simulink model "NUgus_IK"  (R2018a)
settings: Solver=VariableStepAuto  StartTime=0.0  StopTime=inf  RelTol=1e-3
values from neighbouring files (symbols this model uses):
  CM740_acc_bias = 4 * 9.80743    (= 39.22972)    [CM740_init.m]
  CM740_acc_gain = 512 / CM740_acc_centre    [CM740_init.m]
  CM740_gyro_bias = 1600 / 360 * 2 * pi    (= 27.9252680319)    [CM740_init.m]
  CM740_gyro_gain = 512 / CM740_gyro_centre    [CM740_init.m]
  head = [-0.05482228998067195, -0.00010888238321339966, 0.0011712900228573724, 0.41900000000000004]    [comtest.m]
  s = mean(abs(present_speed.data))    [RunServoTest.m]
  torso = [0.0050079703254699804, 0.008880921777563762, 0.1021503146237477, 2.5390000000000006]    [comtest.m]
undefined symbols (not defined in the file or in its folder): floor, X, Y, Z
libraries: sm_lib x211, fl_lib x128, nesl_utility x68
(part 1 of 8)
settings Model: Creator=matt  LastModifiedBy=matt
settings DebuggingCC: UniqueDataStoreMsg=error
settings ExplorerConfigSet: InternalSimMechanicsExplorerSettings="<ExplorerConfiguration><canonicalview>default</canonicalview><AnimationSetting><BasePlaybackSpeed>1.0</BasePlaybackSpeed><PlaybackSpeedFactor>0.125</PlaybackSpeedFactor></AnimationSetting><TilePanel><TileInfo><Tiles Columns=\"1\" Count=\"1\" Rows=\"1\"><Column Weight=\"1\"/><Row Weight=\"1\"/><Tile Height=\"1\" Width=\"1\" X=\"0\" Y=\"0\"/></Tiles></TileInfo><SceneInfo><SceneViewer><BGColor><R>0.800000011920928955</R><G>0.800000011920928955</G><B>0.800000011920928955</B></BGColor><Camera><DoPerspective>off</DoPerspective><Position><X>0.996097398048217064</X><Y>-0.871904325438711214</Y><Z>0.621451067428618886</Z></Position><Center><X>-0.122665475521987533</X><Y>0.224636309977359006</Y><Z>0.297935636755597033</Z></Center><Up><X>-0.160360573572373266</X><Y>0.125250173842771817</Y><Z>0.97907960881426559</Z></Up><ViewLimDist>1</ViewLimDist><YLim>0.594254607494361209</YLim><XLim>0.353738210919678941</XLim></Camera></SceneViewer></SceneInfo></TilePanel><MechEditorPanel><Cameras/><GfxPanelCameraMap/><VideoCreator><PlaybackSpeedRatio>1.0</PlaybackSpeedRatio><FrameRate>30</FrameRate><VideoFormat>Motion JPEG AVI</VideoFormat><FrameSize>auto</FrameSize></VideoCreator></MechEditorPanel></ExplorerConfiguration>"

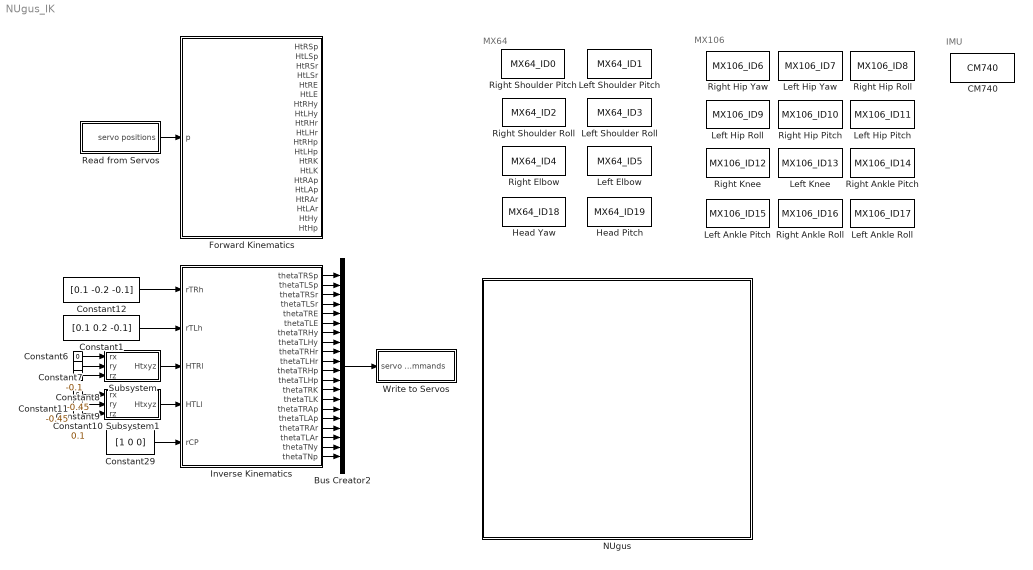
== system NUgus_IK ==
  note: IMU
  note: MX64
  note: MX106
  Bus Creator2 : BusCreator  Inputs=20
  CM740 : DataStoreMemory  DataStoreName=CM740  ReadBeforeWriteMsg=warning  WriteAfterWriteMsg=warning  WriteAfterReadMsg=warning  InitialValue=CM740_default  VectorParams1D=off  ShowAdditionalParam=off  OutDataTypeStr=Bus: CM740_bus
  Constant1 : Constant  Value=[0.1 0.2 -0.1]
  Constant10 : Constant  Value=0.1
  Constant11 : Constant  Value=-0.45
  Constant12 : Constant  Value=[0.1 -0.2 -0.1]
  Constant29 : Constant  Value=[1 0 0]
  Constant6 : Constant  Value=0
  Constant7 : Constant  Value=-0.1
  Constant8 : Constant  Value=-0.45
  Constant9 : Constant  Value=0
  Forward Kinematics : Subsystem
  Head Pitch : DataStoreMemory  DataStoreName=MX64_ID19  ReadBeforeWriteMsg=warning  WriteAfterWriteMsg=warning  WriteAfterReadMsg=warning  InitialValue=MX64_default  VectorParams1D=off  ShowAdditionalParam=off  OutDataTypeStr=Bus: MX64_bus
  Head Yaw : DataStoreMemory  DataStoreName=MX64_ID18  ReadBeforeWriteMsg=warning  WriteAfterWriteMsg=warning  WriteAfterReadMsg=warning  InitialValue=MX64_default  VectorParams1D=off  ShowAdditionalParam=off  OutDataTypeStr=Bus: MX64_bus
  Inverse Kinematics : Subsystem
  Left Ankle Pitch : DataStoreMemory  DataStoreName=MX106_ID15  ReadBeforeWriteMsg=warning  WriteAfterWriteMsg=warning  WriteAfterReadMsg=warning  InitialValue=MX106_default  VectorParams1D=off  ShowAdditionalParam=off  OutDataTypeStr=Bus: MX106_bus
  Left Ankle Roll : DataStoreMemory  DataStoreName=MX106_ID17  ReadBeforeWriteMsg=warning  WriteAfterWriteMsg=warning  WriteAfterReadMsg=warning  InitialValue=MX106_default  VectorParams1D=off  ShowAdditionalParam=off  OutDataTypeStr=Bus: MX106_bus
  Left Elbow : DataStoreMemory  DataStoreName=MX64_ID5  ReadBeforeWriteMsg=warning  WriteAfterWriteMsg=warning  WriteAfterReadMsg=warning  InitialValue=MX64_default  VectorParams1D=off  ShowAdditionalParam=off  OutDataTypeStr=Bus: MX64_bus
  Left Hip Pitch : DataStoreMemory  DataStoreName=MX106_ID11  ReadBeforeWriteMsg=warning  WriteAfterWriteMsg=warning  WriteAfterReadMsg=warning  InitialValue=MX106_default  VectorParams1D=off  ShowAdditionalParam=off  OutDataTypeStr=Bus: MX106_bus
  Left Hip Roll : DataStoreMemory  DataStoreName=MX106_ID9  ReadBeforeWriteMsg=warning  WriteAfterWriteMsg=warning  WriteAfterReadMsg=warning  InitialValue=MX106_default  VectorParams1D=off  ShowAdditionalParam=off  OutDataTypeStr=Bus: MX106_bus
  Left Hip Yaw : DataStoreMemory  DataStoreName=MX106_ID7  ReadBeforeWriteMsg=warning  WriteAfterWriteMsg=warning  WriteAfterReadMsg=warning  InitialValue=MX106_default  VectorParams1D=off  ShowAdditionalParam=off  OutDataTypeStr=Bus: MX106_bus
  Left Knee : DataStoreMemory  DataStoreName=MX106_ID13  ReadBeforeWriteMsg=warning  WriteAfterWriteMsg=warning  WriteAfterReadMsg=warning  InitialValue=MX106_default  VectorParams1D=off  ShowAdditionalParam=off  OutDataTypeStr=Bus: MX106_bus
  Left Shoulder Pitch : DataStoreMemory  DataStoreName=MX64_ID1  ReadBeforeWriteMsg=warning  WriteAfterWriteMsg=warning  WriteAfterReadMsg=warning  InitialValue=MX64_default  VectorParams1D=off  ShowAdditionalParam=off  OutDataTypeStr=Bus: MX64_bus
  Left Shoulder Roll : DataStoreMemory  DataStoreName=MX64_ID3  ReadBeforeWriteMsg=warning  WriteAfterWriteMsg=warning  WriteAfterReadMsg=warning  InitialValue=MX64_default  VectorParams1D=off  ShowAdditionalParam=off  OutDataTypeStr=Bus: MX64_bus
  NUgus : Subsystem
      mask Display: image('./img/NUgus.png');
  Read from Servos : Subsystem
  Right Ankle Pitch : DataStoreMemory  DataStoreName=MX106_ID14  ReadBeforeWriteMsg=warning  WriteAfterWriteMsg=warning  WriteAfterReadMsg=warning  InitialValue=MX106_default  VectorParams1D=off  ShowAdditionalParam=off  OutDataTypeStr=Bus: MX106_bus
  Right Ankle Roll : DataStoreMemory  DataStoreName=MX106_ID16  ReadBeforeWriteMsg=warning  WriteAfterWriteMsg=warning  WriteAfterReadMsg=warning  InitialValue=MX106_default  VectorParams1D=off  ShowAdditionalParam=off  OutDataTypeStr=Bus: MX106_bus
  Right Elbow : DataStoreMemory  DataStoreName=MX64_ID4  ReadBeforeWriteMsg=warning  WriteAfterWriteMsg=warning  WriteAfterReadMsg=warning  InitialValue=MX64_default  VectorParams1D=off  ShowAdditionalParam=off  OutDataTypeStr=Bus: MX64_bus
  Right Hip Pitch : DataStoreMemory  DataStoreName=MX106_ID10  ReadBeforeWriteMsg=warning  WriteAfterWriteMsg=warning  WriteAfterReadMsg=warning  InitialValue=MX106_default  VectorParams1D=off  ShowAdditionalParam=off  OutDataTypeStr=Bus: MX106_bus
  Right Hip Roll : DataStoreMemory  DataStoreName=MX106_ID8  ReadBeforeWriteMsg=warning  WriteAfterWriteMsg=warning  WriteAfterReadMsg=warning  InitialValue=MX106_default  VectorParams1D=off  ShowAdditionalParam=off  OutDataTypeStr=Bus: MX106_bus
  Right Hip Yaw : DataStoreMemory  DataStoreName=MX106_ID6  InitialValue=MX106_default  VectorParams1D=off  ShowAdditionalParam=off  OutDataTypeStr=Bus: MX106_bus
  Right Knee : DataStoreMemory  DataStoreName=MX106_ID12  ReadBeforeWriteMsg=warning  WriteAfterWriteMsg=warning  WriteAfterReadMsg=warning  InitialValue=MX106_default  VectorParams1D=off  ShowAdditionalParam=off  OutDataTypeStr=Bus: MX106_bus
  Right Shoulder Pitch : DataStoreMemory  DataStoreName=MX64_ID0  ReadBeforeWriteMsg=warning  WriteAfterWriteMsg=warning  WriteAfterReadMsg=warning  InitialValue=MX64_default  VectorParams1D=off  ShowAdditionalParam=off  OutDataTypeStr=Bus: MX64_bus
  Right Shoulder Roll : DataStoreMemory  DataStoreName=MX64_ID2  ReadBeforeWriteMsg=warning  WriteAfterWriteMsg=warning  WriteAfterReadMsg=warning  InitialValue=MX64_default  VectorParams1D=off  ShowAdditionalParam=off  OutDataTypeStr=Bus: MX64_bus
  Subsystem : Subsystem
  Subsystem1 : Subsystem
  Write to Servos : Subsystem
  wires:
  Inverse Kinematics/1(thetaTRSp) -> Bus Creator2/1
  Inverse Kinematics/2(thetaTLSp) -> Bus Creator2/2
  Inverse Kinematics/3(thetaTRSr) -> Bus Creator2/3
  Inverse Kinematics/4(thetaTLSr) -> Bus Creator2/4
  Inverse Kinematics/5(thetaTRE) -> Bus Creator2/5
  Inverse Kinematics/6(thetaTLE) -> Bus Creator2/6
  Inverse Kinematics/7(thetaTRHy) -> Bus Creator2/7
  Inverse Kinematics/8(thetaTLHy) -> Bus Creator2/8
  Inverse Kinematics/9(thetaTRHr) -> Bus Creator2/9
  Inverse Kinematics/10(thetaTLHr) -> Bus Creator2/10
  Inverse Kinematics/11(thetaTRHp) -> Bus Creator2/11
  Inverse Kinematics/12(thetaTLHp) -> Bus Creator2/12
  Inverse Kinematics/13(thetaTRK) -> Bus Creator2/13
  Inverse Kinematics/14(thetaTLK) -> Bus Creator2/14
  Inverse Kinematics/15(thetaTRAp) -> Bus Creator2/15
  Inverse Kinematics/16(thetaTLAp) -> Bus Creator2/16
  Inverse Kinematics/17(thetaTRAr) -> Bus Creator2/17
  Inverse Kinematics/18(thetaTLAr) -> Bus Creator2/18
  Inverse Kinematics/19(thetaTNy) -> Bus Creator2/19
  Inverse Kinematics/20(thetaTNp) -> Bus Creator2/20
  Bus Creator2/1 -> Write to Servos/1(servo commands)
  Constant12/1 -> Inverse Kinematics/1(rTRh)
  Constant1/1 -> Inverse Kinematics/2(rTLh)
  Constant29/1 -> Inverse Kinematics/5(rCP)
  Constant7/1 -> Subsystem/2(ry)
  Constant8/1 -> Subsystem/3(rz)
  Constant6/1 -> Subsystem/1(rx)
  Subsystem/1(Htxyz) -> Inverse Kinematics/3(HTRl)
  Constant11/1 -> Subsystem1/3(rz)
  Constant9/1 -> Subsystem1/1(rx)
  Constant10/1 -> Subsystem1/2(ry)
  Subsystem1/1(Htxyz) -> Inverse Kinematics/4(HTLl)
  Read from Servos/1(servo positions) -> Forward Kinematics/1(p)

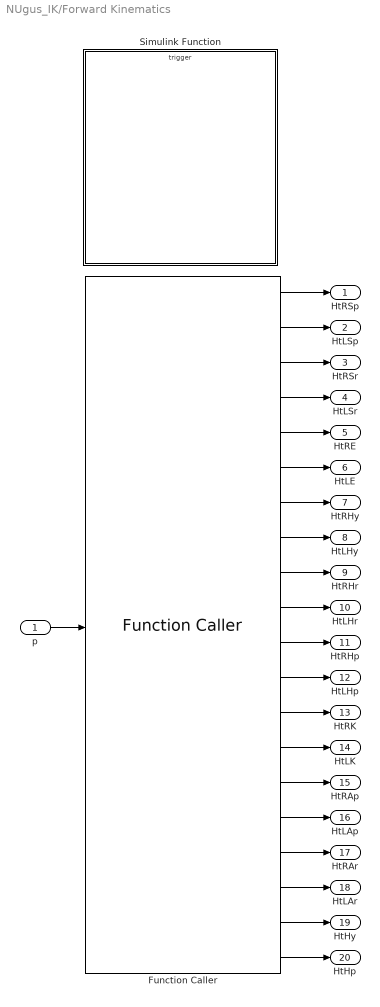
== system NUgus_IK/Forward Kinematics ==
  p : Inport
  Function Caller : FunctionCaller  FunctionPrototype=[HtRSp,HtLSp,HtRSr,HtLSr,HtRE,HtLE,HtRHy,HtLHy,HtRHr,HtLHr,HtRHp,HtLHp,HtRK,HtLK,HtRAp,HtLAp,HtRAr,HtLAr,HtHy,HtHp] = FK(p)  InputArgumentSpecifications=double([1 1 1 1 1 1 1 1 1 1 1 1 1 1 1 1 1 1 1 1])
  Simulink Function : Subsystem  TreatAsAtomicUnit=on
  HtRSp : Outport
  HtLSp : Outport  Port=2
  HtRSr : Outport  Port=3
  HtLSr : Outport  Port=4
  HtRE : Outport  Port=5
  HtLE : Outport  Port=6
  HtRHy : Outport  Port=7
  HtLHy : Outport  Port=8
  HtRHr : Outport  Port=9
  HtLHr : Outport  Port=10
  HtRHp : Outport  Port=11
  HtLHp : Outport  Port=12
  HtRK : Outport  Port=13
  HtLK : Outport  Port=14
  HtRAp : Outport  Port=15
  HtLAp : Outport  Port=16
  HtRAr : Outport  Port=17
  HtLAr : Outport  Port=18
  HtHy : Outport  Port=19
  HtHp : Outport  Port=20
  wires:
  Function Caller/2 -> HtLSp/1
  Function Caller/1 -> HtRSp/1
  Function Caller/3 -> HtRSr/1
  Function Caller/4 -> HtLSr/1
  Function Caller/5 -> HtRE/1
  Function Caller/6 -> HtLE/1
  Function Caller/7 -> HtRHy/1
  Function Caller/8 -> HtLHy/1
  Function Caller/9 -> HtRHr/1
  Function Caller/10 -> HtLHr/1
  Function Caller/11 -> HtRHp/1
  Function Caller/12 -> HtLHp/1
  Function Caller/13 -> HtRK/1
  Function Caller/14 -> HtLK/1
  Function Caller/15 -> HtRAp/1
  Function Caller/16 -> HtLAp/1
  Function Caller/17 -> HtRAr/1
  Function Caller/18 -> HtLAr/1
  Function Caller/19 -> HtHy/1
  Function Caller/20 -> HtHp/1
  p/1 -> Function Caller/1

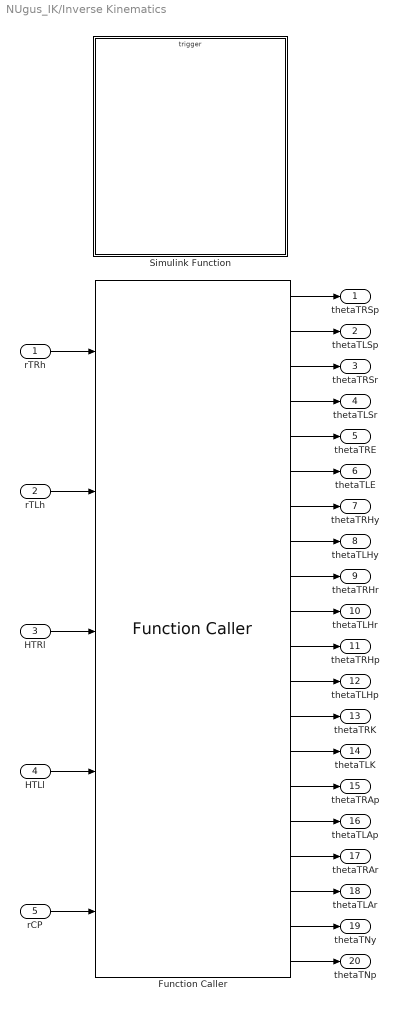
== system NUgus_IK/Inverse Kinematics ==
  rTRh : Inport
  rTLh : Inport  Port=2
  HTRl : Inport  Port=3
  HTLl : Inport  Port=4
  rCP : Inport  Port=5
  Function Caller : FunctionCaller  FunctionPrototype=[thetaTRSp,thetaTLSp,thetaTRSr,thetaTLSr,thetaTRE,thetaTLE,thetaTRHy,thetaTLHy,thetaTRHr,thetaTLHr,thetaTRHp,thetaTLHp,thetaTRK,thetaTLK,thetaTRAp,thetaTLAp,thetaTRAr,thetaTLAr,thetaTNy,thetaTNp] = IK(rTRh,rTLh,HTRl,HTLl,rCP)
  Simulink Function : Subsystem  TreatAsAtomicUnit=on
  thetaTRSp : Outport
  thetaTLSp : Outport  Port=2
  thetaTRSr : Outport  Port=3
  thetaTLSr : Outport  Port=4
  thetaTRE : Outport  Port=5
  thetaTLE : Outport  Port=6
  thetaTRHy : Outport  Port=7
  thetaTLHy : Outport  Port=8
  thetaTRHr : Outport  Port=9
  thetaTLHr : Outport  Port=10
  thetaTRHp : Outport  Port=11
  thetaTLHp : Outport  Port=12
  thetaTRK : Outport  Port=13
  thetaTLK : Outport  Port=14
  thetaTRAp : Outport  Port=15
  thetaTLAp : Outport  Port=16
  thetaTRAr : Outport  Port=17
  thetaTLAr : Outport  Port=18
  thetaTNy : Outport  Port=19
  thetaTNp : Outport  Port=20
  wires:
  Function Caller/2 -> thetaTLSp/1
  Function Caller/1 -> thetaTRSp/1
  Function Caller/3 -> thetaTRSr/1
  Function Caller/4 -> thetaTLSr/1
  Function Caller/5 -> thetaTRE/1
  Function Caller/6 -> thetaTLE/1
  Function Caller/7 -> thetaTRHy/1
  Function Caller/8 -> thetaTLHy/1
  Function Caller/9 -> thetaTRHr/1
  Function Caller/10 -> thetaTLHr/1
  Function Caller/11 -> thetaTRHp/1
  Function Caller/12 -> thetaTLHp/1
  Function Caller/13 -> thetaTRK/1
  Function Caller/14 -> thetaTLK/1
  Function Caller/15 -> thetaTRAp/1
  Function Caller/16 -> thetaTLAp/1
  Function Caller/17 -> thetaTRAr/1
  Function Caller/18 -> thetaTLAr/1
  Function Caller/19 -> thetaTNy/1
  Function Caller/20 -> thetaTNp/1
  rTRh/1 -> Function Caller/1
  rTLh/1 -> Function Caller/2
  HTRl/1 -> Function Caller/3
  HTLl/1 -> Function Caller/4
  rCP/1 -> Function Caller/5

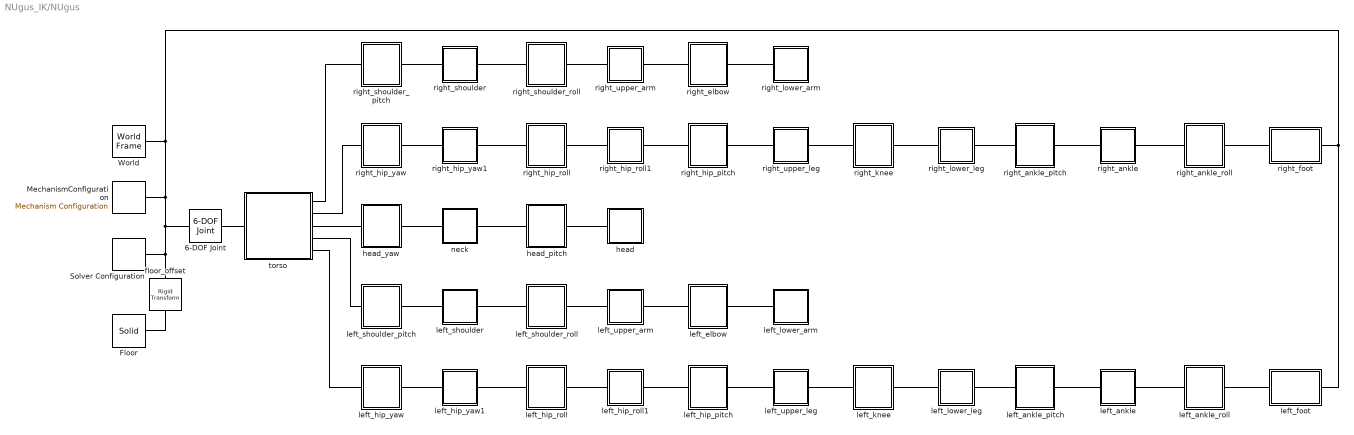
== system NUgus_IK/NUgus ==
  6-DOF Joint : sm_lib/Joints/6-DOF Joint  SenseConstraintForce=off  SenseConstraintForceX=off  SenseConstraintForceY=off  SenseConstraintForceZ=off  SenseConstraintTorque=off  SenseConstraintTorqueX=off  SenseConstraintTorqueY=off  SenseConstraintTorqueZ=off  SenseTotalForce=off  SenseTotalForceX=off  SenseTotalForceY=off  SenseTotalForceZ=off  SenseTotalTorque=off  SenseTotalTorqueX=off  SenseTotalTorqueY=off  SenseTotalTorqueZ=off  CompositeWrenchDir=FollowerOnBase  CompositeWrenchFrame=BaseFrame  PxEquilibriumPosition=0  PxEquilibriumPositionUnits=m  PxSpringStiffness=0  PxSpringStiffnessUnits=N/m  PxDampingCoefficient=0  PxDampingCoefficientUnits=N/(m/s)  PxTorqueActuationMode=NoTorque  PxMotionActuationMode=ComputedMotion  PxSensePosition=off  PxSenseVelocity=off  PxSenseAcceleration=off  PxSenseTorqueForce=off  PxPositionTargetSpecify=off  PxPositionTargetPriority=High  PxPositionTargetValue=0  PxPositionTargetValueUnits=m  PxVelocityTargetSpecify=off  PxVelocityTargetPriority=High  PxVelocityTargetValue=0  PxVelocityTargetValueUnits=m/s  PyEquilibriumPosition=0  PyEquilibriumPositionUnits=m  PySpringStiffness=0  PySpringStiffnessUnits=N/m  PyDampingCoefficient=0  PyDampingCoefficientUnits=N/(m/s)  PyTorqueActuationMode=NoTorque  PyMotionActuationMode=ComputedMotion  PySensePosition=off  PySenseVelocity=off  PySenseAcceleration=off  PySenseTorqueForce=off  PyPositionTargetSpecify=off  PyPositionTargetPriority=High  PyPositionTargetValue=0  PyPositionTargetValueUnits=m  PyVelocityTargetSpecify=off  PyVelocityTargetPriority=High  PyVelocityTargetValue=0  PyVelocityTargetValueUnits=m/s  PzEquilibriumPosition=0  PzEquilibriumPositionUnits=m  PzSpringStiffness=0  PzSpringStiffnessUnits=N/m  PzDampingCoefficient=0  PzDampingCoefficientUnits=N/(m/s)  PzTorqueActuationMode=NoTorque  PzMotionActuationMode=ComputedMotion  PzSensePosition=off  PzSenseVelocity=off  PzSenseAcceleration=off  PzSenseTorqueForce=off  PzPositionTargetSpecify=on  PzPositionTargetPriority=High  PzPositionTargetValue=0.52+floor.depth  PzPositionTargetValueUnits=m  PzVelocityTargetSpecify=off  PzVelocityTargetPriority=High  PzVelocityTargetValue=0  PzVelocityTargetValueUnits=m/s  SphDefPosRotationMethod=None  SphDefPosRotationAngleUnits=deg  SphDefPosRotationStandardAxis=+Z  SphDefPosRotationAngle=0.0  SphDefPosRotationArbitraryAxis=[0 0 1]  SphDefPosFollAlignAxisA=+X  SphDefPosBaseAlignAxisA=+Y  SphDefPosFollAlignAxisB=+Y  SphDefPosBaseAlignAxisB=+Z  SphDefPosRotationSequenceAxes=FollowerAxes  SphDefPosRotationSequence=XYX  SphDefPosRotationSequenceAngles=[0 0 0]  SphDefPosRotationSequenceAnglesUnits=deg  SphDefPosRotationMatrix=[1 0 0; 0 1 0; 0 0 1]  SphEqPosRotationMethod=None  SphEqPosRotationAngleUnits=deg  SphEqPosRotationStandardAxis=+Z  SphEqPosRotationAngle=0.0  SphEqPosRotationArbitraryAxis=[0 0 1]  SphEqPosFollAlignAxisA=+X  SphEqPosBaseAlignAxisA=+Y  SphEqPosFollAlignAxisB=+Y  SphEqPosBaseAlignAxisB=+Z  SphEqPosRotationSequenceAxes=FollowerAxes  SphEqPosRotationSequence=XYX  SphEqPosRotationSequenceAngles=[0 0 0]  SphEqPosRotationSequenceAnglesUnits=deg  SphEqPosRotationMatrix=[1 0 0; 0 1 0; 0 0 1]  SphSpringStiffness=0  SphSpringStiffnessUnits=N*m/deg  SphDampingCoefficient=0  SphDampingCoefficientUnits=N*m/(deg/s)  SphActuateTorqueX=off  SphActuateTorqueY=off  SphActuateTorqueZ=off  SphActuateTorque=off  SphTorqueActuationMode=NoTorque  SphMotionActuationMode=ComputedMotion  SphActuationFrame=BaseFrame  SphSensePosition=off  SphSenseVelocityX=off  SphSenseVelocityY=off  SphSenseVelocityZ=off  SphSenseVelocity=off  SphSenseAccelerationX=off  SphSenseAccelerationY=off  SphSenseAccelerationZ=off  SphSenseAcceleration=off  SphSenseTorqueX=off  SphSenseTorqueY=off  SphSenseTorqueZ=off  SphSenseTorqueForce=off  SphSensingFrame=BaseFrame  SphPositionTargetRotationMethod=None  SphPositionTargetRotationAngleUnits=deg  SphPositionTargetRotationStandardAxis=+Z  SphPositionTargetRotationAngle=0.0  SphPositionTargetRotationArbitraryAxis=[0 0 1]  SphPositionTargetFollAlignAxisA=+X  SphPositionTargetBaseAlignAxisA=+Y  SphPositionTargetFollAlignAxisB=+Y  SphPositionTargetBaseAlignAxisB=+Z  SphPositionTargetRotationSequenceAxes=FollowerAxes  SphPositionTargetRotationSequence=XYX  SphPositionTargetRotationSequenceAngles=[0 0 0]  SphPositionTargetRotationSequenceAnglesUnits=deg  SphPositionTargetRotationMatrix=[1 0 0; 0 1 0; 0 0 1]  SphPositionTargetSpecify=off  SphPositionTargetPriority=High  SphVelocityTargetValue=[0 0 0]  SphVelocityTargetValueUnits=deg/s  SphVelocityTargetSpecify=off  SphVelocityTargetPriority=High  SphVelocityTargetInFollowerFrame=on
  Floor : sm_lib/Body Elements/Solid  InertiaType=CalculateFromGeometry  Mass=1  MassUnits=kg  CenterOfMass=[0 0 0]  CenterOfMassUnits=m  MomentsOfInertia=[1 1 1]  MomentsOfInertiaUnits=kg*m^2  ProductsOfInertia=[0 0 0]  ProductsOfInertiaUnits=kg*m^2  DensityBased=on  Density=1000  DensityUnits=kg/m^3  DoExposeReferenceFrame=on  SerializedFrames=<Frames/>  GraphicType=FromGeometry  MarkerShape=Frame  MarkerSize=10  GraphicVisPropType=SimpleVisualProperties  GraphicDiffuseColor=[0.972549 0.972549 0.972549]  GraphicSpecularColor=[0.3 0.3 0.3 1.0]  GraphicAmbientColor=[0.20 0.20 0.20 1.0]  GraphicEmissiveColor=[0.0 0.0 0.0 1.0]  GraphicShininess=30  GraphicOpacity=0.6  GeometryShape=Brick  RectangleSize=[1 1]  RectangleSizeUnits=m  BrickDimensions=[floor.length floor.width floor.depth]  BrickDimensionUnits=m  CylinderRadius=1  CylinderRadiusUnits=m  CylinderLength=1  CylinderLengthUnits=m  SphereRadius=1  SphereRadiusUnits=m  EllipsoidRadii=[1 1 1]  EllipsoidRadiiUnits=m  ExtrusionCrossSection=[1 1; -1 1; -1 -1; 1 -1]  ExtrusionCrossSectionUnits=m  ExtrusionLength=1  ExtrusionLengthUnits=m  PolygonNumSides=3  PolygonOuterRadius=1  PolygonOuterRadiusUnits=m  ExtGeomFileType=STEP  ExtGeomFileUnits=m  RevolutionCrossSection=[1 1; 1 -1; 2 -1; 2 1]  RevolutionCrossSectionUnits=m  RevolutionExtent=Full  RevolutionAngle=180  RevolutionAngleUnits=deg
  MechanismConfiguration : sm_lib/Utilities/Mechanism Configuration  UniformGravity=Constant  GravityVector=[0 0 -9.80665]  GravityUnits=m/s^2  LinearizationDelta=0.001
  Solver Configuration : nesl_utility/Solver Configuration  PhysicalDomain=network_engine_domain  SubClassName=solver  LeftPortType=input  RightPortType=generic  Tones=[]  Harmonics=[]  SimulateNoise=off  Profile=off  UseLocalSampling=off  EnableSwitchedLinearOptims=on  FrequencyDomain=off  UseCCode=off  RelTol=0.001  AbsTol=1e-06  MinStep=1e-09  ToWorkspace=off  RevertToSquareIcSolve=off  NumHomotopyIterations=100  PhasorMode=off  PhasorModeNumHarmonics=1  DoDC=off  ResidualTolerance=1e-09  UseLocalSolver=off  LocalSolverChoice=NE_BACKWARD_EULER_ADVANCER  LocalSolverSampleTime=0.001  DoFixedCost=off  MaxNonlinIter=3  MaxModeIter=2  LinearAlgebra=Sparse  EquationFormulation=NE_TIME_EF  DelaysMemoryBudget=1024  AutomaticFiltering=on  FilteringTimeConstant=0.001
  World : sm_lib/Frames and Transforms/World Frame
  floor_offset : sm_lib/Frames and Transforms/Rigid Transform  TranslationMethod=Cartesian  TranslationStandardOffset=0  TranslationLengthUnit=m  TranslationStandardAxis=+Z  TranslationCartesianOffset=[0 0 floor.depth/2]  TranslationROffset=0  TranslationROffsetUnits=m  TranslationZOffset=0  TranslationZOffsetUnits=m  TranslationThetaOffset=0  TranslationThetaOffsetUnits=deg  RotationMethod=None  RotationAngleUnits=deg  RotationStandardAxis=+Z  RotationAngle=0.0  RotationArbitraryAxis=[0 0 1]  FollAlignAxisA=+X  BaseAlignAxisA=+Y  FollAlignAxisB=+Y  BaseAlignAxisB=+Z  RotationSequenceAxes=FollowerAxes  RotationSequence=XYX  RotationSequenceAngles=[0 0 0]  RotationSequenceAnglesUnits=deg  RotationMatrix=[1 0 0; 0 1 0; 0 0 1]
  head : Subsystem
  head_pitch : Subsystem
      mask Display: image('./img/MX64.png');
  head_yaw : Subsystem
      mask Display: image('./img/MX64.png');
  left_ankle : Subsystem
  left_ankle_pitch : Subsystem
      mask Display: image('./img/MX106.png');
  left_ankle_roll : Subsystem
      mask Display: image('./img/MX106.png');
  left_elbow : Subsystem
      mask Display: image('./img/MX64.png');
  left_foot : Subsystem
  left_hip_pitch : Subsystem
      mask Display: image('./img/MX106.png');
  left_hip_roll : Subsystem
      mask Display: image('./img/MX106.png');
  left_hip_roll1 : Subsystem
  left_hip_yaw : Subsystem
      mask Display: image('./img/MX106.png');
  left_hip_yaw1 : Subsystem
  left_knee : Subsystem
      mask Display: image('./img/MX106.png');
  left_lower_arm : Subsystem
  left_lower_leg : Subsystem
  left_shoulder : Subsystem
  left_shoulder_pitch : Subsystem
      mask Display: image('./img/MX64.png');
  left_shoulder_roll : Subsystem
      mask Display: image('./img/MX64.png');
  left_upper_arm : Subsystem
  left_upper_leg : Subsystem
  neck : Subsystem
  right_ankle : Subsystem
  right_ankle_pitch : Subsystem
      mask Display: image('./img/MX106.png');
  right_ankle_roll : Subsystem
      mask Display: image('./img/MX106.png');
  right_elbow : Subsystem
      mask Display: image('./img/MX64.png');
  right_foot : Subsystem
  right_hip_pitch : Subsystem
      mask Display: image('./img/MX106.png');
  right_hip_roll : Subsystem
      mask Display: image('./img/MX106.png');
  right_hip_roll1 : Subsystem
  right_hip_yaw : Subsystem
      mask Display: image('./img/MX106.png');
  right_hip_yaw1 : Subsystem
  right_knee : Subsystem
      mask Display: image('./img/MX106.png');
  right_lower_arm : Subsystem
  right_lower_leg : Subsystem
  right_shoulder : Subsystem
  right_shoulder_pitch : Subsystem
      mask Display: image('./img/MX64.png');
  right_shoulder_roll : Subsystem
      mask Display: image('./img/MX64.png');
  right_upper_arm : Subsystem
  right_upper_leg : Subsystem
  torso : Subsystem
  connections:
  right_ankle_roll/LConn1 -- right_ankle/RConn1
  left_elbow/RConn1 -- left_lower_arm/LConn1
  left_knee/RConn1 -- left_lower_leg/LConn1
  left_hip_roll/LConn1 -- left_hip_yaw1/RConn1
  left_hip_yaw/RConn1 -- left_hip_yaw1/LConn1
  torso/RConn3 -- head_yaw/LConn1
  right_shoulder_roll/LConn1 -- right_shoulder/RConn1
  right_hip_pitch/LConn1 -- right_hip_roll1/RConn1
  right_hip_yaw1/RConn1 -- right_hip_roll/LConn1
  head_pitch/LConn1 -- neck/RConn1
  6-DOF Joint/RConn1 -- torso/LConn1
  Floor/RConn1 -- floor_offset/RConn1
  right_lower_arm/LConn1 -- right_elbow/RConn1
  head/LConn1 -- head_pitch/RConn1
  left_shoulder/RConn1 -- left_shoulder_roll/LConn1
  left_hip_pitch/RConn1 -- left_upper_leg/LConn1
  left_foot/LConn1 -- left_ankle_roll/RConn1
  torso/RConn1 -- right_shoulder_pitch/LConn1
  right_hip_pitch/RConn1 -- right_upper_leg/LConn1
  right_hip_yaw/LConn1 -- torso/RConn2
  left_shoulder_pitch/LConn1 -- torso/RConn4
  left_ankle_pitch/RConn1 -- left_ankle/LConn1
  left_ankle_pitch/LConn1 -- left_lower_leg/RConn1
  left_knee/LConn1 -- left_upper_leg/RConn1
  left_hip_roll/RConn1 -- left_hip_roll1/LConn1
  MechanismConfiguration/RConn1 -- left_foot/RConn1 -- right_foot/RConn1 -- World/RConn1 -- 6-DOF Joint/LConn1 -- floor_offset/LConn1 -- Solver Configuration/RConn1
  left_upper_arm/LConn1 -- left_shoulder_roll/RConn1
  left_shoulder_pitch/RConn1 -- left_shoulder/LConn1
  left_ankle_roll/LConn1 -- left_ankle/RConn1
  right_ankle_pitch/RConn1 -- right_ankle/LConn1
  right_ankle_pitch/LConn1 -- right_lower_leg/RConn1
  neck/LConn1 -- head_yaw/RConn1
  right_knee/RConn1 -- right_lower_leg/LConn1
  right_ankle_roll/RConn1 -- right_foot/LConn1
  right_knee/LConn1 -- right_upper_leg/RConn1
  right_hip_roll1/LConn1 -- right_hip_roll/RConn1
  right_shoulder_pitch/RConn1 -- right_shoulder/LConn1
  right_elbow/LConn1 -- right_upper_arm/RConn1
  right_hip_yaw/RConn1 -- right_hip_yaw1/LConn1
  left_elbow/LConn1 -- left_upper_arm/RConn1
  left_hip_roll1/RConn1 -- left_hip_pitch/LConn1
  torso/RConn5 -- left_hip_yaw/LConn1
  right_shoulder_roll/RConn1 -- right_upper_arm/LConn1

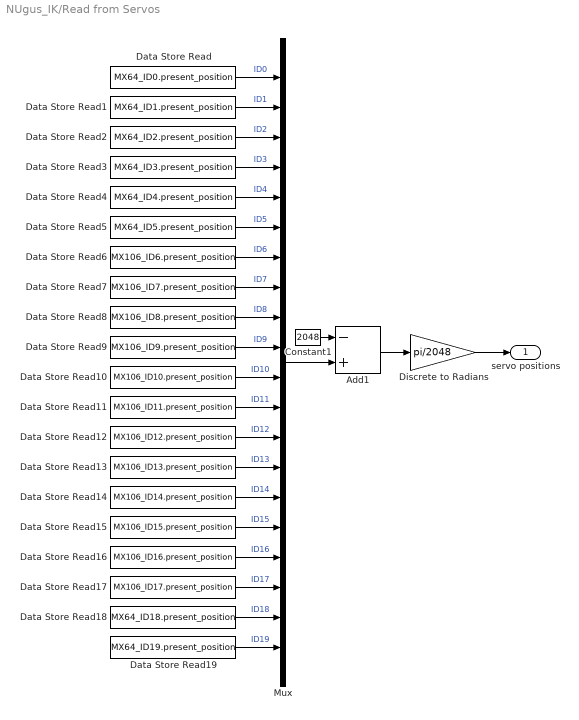
== system NUgus_IK/Read from Servos ==
  Add1 : Sum  Inputs=-+  OutDataTypeStr=double
  Constant1 : Constant  Value=2048
  Data Store Read : DataStoreRead  DataStoreName=MX64_ID0  DataStoreElements=MX64_ID0.present_position
  Data Store Read1 : DataStoreRead  DataStoreName=MX64_ID1  DataStoreElements=MX64_ID1.present_position
  Data Store Read10 : DataStoreRead  DataStoreName=MX106_ID10  DataStoreElements=MX106_ID10.present_position
  Data Store Read11 : DataStoreRead  DataStoreName=MX106_ID11  DataStoreElements=MX106_ID11.present_position
  Data Store Read12 : DataStoreRead  DataStoreName=MX106_ID12  DataStoreElements=MX106_ID12.present_position
  Data Store Read13 : DataStoreRead  DataStoreName=MX106_ID13  DataStoreElements=MX106_ID13.present_position
  Data Store Read14 : DataStoreRead  DataStoreName=MX106_ID14  DataStoreElements=MX106_ID14.present_position
  Data Store Read15 : DataStoreRead  DataStoreName=MX106_ID15  DataStoreElements=MX106_ID15.present_position
  Data Store Read16 : DataStoreRead  DataStoreName=MX106_ID16  DataStoreElements=MX106_ID16.present_position
  Data Store Read17 : DataStoreRead  DataStoreName=MX106_ID17  DataStoreElements=MX106_ID17.present_position
  Data Store Read18 : DataStoreRead  DataStoreName=MX64_ID18  DataStoreElements=MX64_ID18.present_position
  Data Store Read19 : DataStoreRead  DataStoreName=MX64_ID19  DataStoreElements=MX64_ID19.present_position
  Data Store Read2 : DataStoreRead  DataStoreName=MX64_ID2  DataStoreElements=MX64_ID2.present_position
  Data Store Read3 : DataStoreRead  DataStoreName=MX64_ID3  DataStoreElements=MX64_ID3.present_position
  Data Store Read4 : DataStoreRead  DataStoreName=MX64_ID4  DataStoreElements=MX64_ID4.present_position
  Data Store Read5 : DataStoreRead  DataStoreName=MX64_ID5  DataStoreElements=MX64_ID5.present_position
  Data Store Read6 : DataStoreRead  DataStoreName=MX106_ID6  DataStoreElements=MX106_ID6.present_position
  Data Store Read7 : DataStoreRead  DataStoreName=MX106_ID7  DataStoreElements=MX106_ID7.present_position
  Data Store Read8 : DataStoreRead  DataStoreName=MX106_ID8  DataStoreElements=MX106_ID8.present_position
  Data Store Read9 : DataStoreRead  DataStoreName=MX106_ID9  DataStoreElements=MX106_ID9.present_position
  Discrete to Radians : Gain  Gain=pi/2048  SaturateOnIntegerOverflow=on  OutDataTypeStr=Inherit: Same as input
  Mux : Mux  Inputs=20
  servo positions : Outport  PortDimensions=20
  wires:
  Data Store Read19/1 -> Mux/20  "ID19"
  Data Store Read18/1 -> Mux/19  "ID18"
  Data Store Read17/1 -> Mux/18  "ID17"
  Data Store Read/1 -> Mux/1  "ID0"
  Data Store Read1/1 -> Mux/2  "ID1"
  Data Store Read2/1 -> Mux/3  "ID2"
  Data Store Read3/1 -> Mux/4  "ID3"
  Data Store Read4/1 -> Mux/5  "ID4"
  Data Store Read5/1 -> Mux/6  "ID5"
  Data Store Read6/1 -> Mux/7  "ID6"
  Data Store Read7/1 -> Mux/8  "ID7"
  Data Store Read8/1 -> Mux/9  "ID8"
  Data Store Read9/1 -> Mux/10  "ID9"
  Data Store Read10/1 -> Mux/11  "ID10"
  Data Store Read11/1 -> Mux/12  "ID11"
  Data Store Read12/1 -> Mux/13  "ID12"
  Data Store Read13/1 -> Mux/14  "ID13"
  Data Store Read14/1 -> Mux/15  "ID14"
  Data Store Read15/1 -> Mux/16  "ID15"
  Data Store Read16/1 -> Mux/17  "ID16"
  Mux/1 -> Add1/2
  Constant1/1 -> Add1/1
  Add1/1 -> Discrete to Radians/1
  Discrete to Radians/1 -> servo positions/1

== system NUgus_IK/Subsystem ==
  rx : Inport
  ry : Inport  Port=2
  rz : Inport  Port=3
  Bus Creator3 : BusCreator  Inputs=4
  Bus to Vector2 : BusToVector
  Constant : Constant
  Constant9 : Constant  Value=[1 0 0; 0 1 0; 0 0 1; 0 0 0]
  Matrix Concatenate : Concatenate  Mode=Multidimensional array  ConcatenateDimension=2
  Htxyz : Outport
  wires:
  Bus to Vector2/1 -> Matrix Concatenate/2
  ry/1 -> Bus Creator3/2
  Bus Creator3/1 -> Bus to Vector2/1
  Matrix Concatenate/1 -> Htxyz/1
  rx/1 -> Bus Creator3/1
  rz/1 -> Bus Creator3/3
  Constant9/1 -> Matrix Concatenate/1
  Constant/1 -> Bus Creator3/4

== system NUgus_IK/Subsystem1 ==
  rx : Inport
  ry : Inport  Port=2
  rz : Inport  Port=3
  Bus Creator3 : BusCreator  Inputs=4
  Bus to Vector2 : BusToVector
  Constant : Constant
  Constant9 : Constant  Value=[1 0 0; 0 1 0; 0 0 1; 0 0 0]
  Matrix Concatenate : Concatenate  Mode=Multidimensional array  ConcatenateDimension=2
  Htxyz : Outport
  wires:
  Bus to Vector2/1 -> Matrix Concatenate/2
  ry/1 -> Bus Creator3/2
  Bus Creator3/1 -> Bus to Vector2/1
  Matrix Concatenate/1 -> Htxyz/1
  rx/1 -> Bus Creator3/1
  rz/1 -> Bus Creator3/3
  Constant9/1 -> Matrix Concatenate/1
  Constant/1 -> Bus Creator3/4

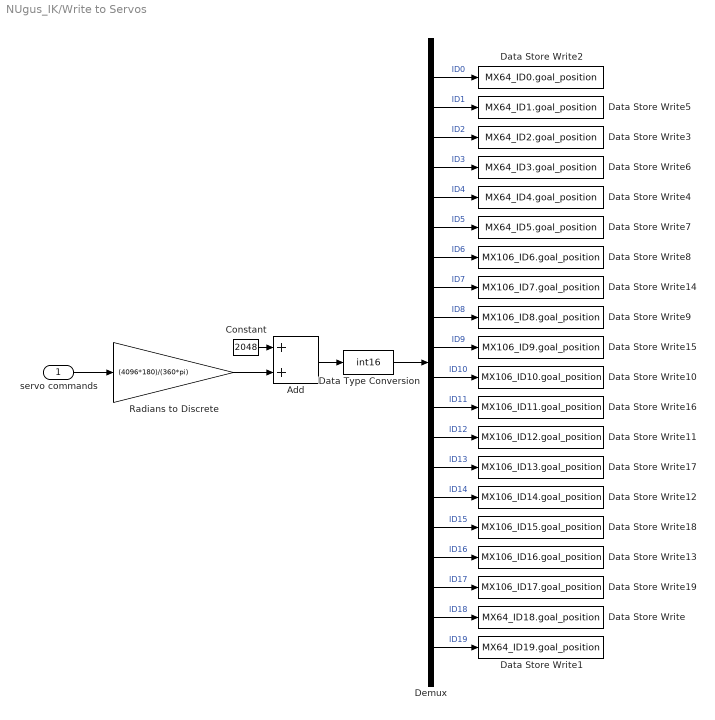
== system NUgus_IK/Write to Servos ==
  servo commands : Inport  PortDimensions=20
  Add : Sum
  Constant : Constant  Value=2048
  Data Store Write : DataStoreWrite  DataStoreName=MX64_ID18  DataStoreElements=MX64_ID18.goal_position
  Data Store Write1 : DataStoreWrite  DataStoreName=MX64_ID19  DataStoreElements=MX64_ID19.goal_position
  Data Store Write10 : DataStoreWrite  DataStoreName=MX106_ID10  DataStoreElements=MX106_ID10.goal_position
  Data Store Write11 : DataStoreWrite  DataStoreName=MX106_ID12  DataStoreElements=MX106_ID12.goal_position
  Data Store Write12 : DataStoreWrite  DataStoreName=MX106_ID14  DataStoreElements=MX106_ID14.goal_position
  Data Store Write13 : DataStoreWrite  DataStoreName=MX106_ID16  DataStoreElements=MX106_ID16.goal_position
  Data Store Write14 : DataStoreWrite  DataStoreName=MX106_ID7  DataStoreElements=MX106_ID7.goal_position
  Data Store Write15 : DataStoreWrite  DataStoreName=MX106_ID9  DataStoreElements=MX106_ID9.goal_position
  Data Store Write16 : DataStoreWrite  DataStoreName=MX106_ID11  DataStoreElements=MX106_ID11.goal_position
  Data Store Write17 : DataStoreWrite  DataStoreName=MX106_ID13  DataStoreElements=MX106_ID13.goal_position
  Data Store Write18 : DataStoreWrite  DataStoreName=MX106_ID15  DataStoreElements=MX106_ID15.goal_position
  Data Store Write19 : DataStoreWrite  DataStoreName=MX106_ID17  DataStoreElements=MX106_ID17.goal_position
  Data Store Write2 : DataStoreWrite  DataStoreName=MX64_ID0  DataStoreElements=MX64_ID0.goal_position
  Data Store Write3 : DataStoreWrite  DataStoreName=MX64_ID2  DataStoreElements=MX64_ID2.goal_position
  Data Store Write4 : DataStoreWrite  DataStoreName=MX64_ID4  DataStoreElements=MX64_ID4.goal_position
  Data Store Write5 : DataStoreWrite  DataStoreName=MX64_ID1  DataStoreElements=MX64_ID1.goal_position
  Data Store Write6 : DataStoreWrite  DataStoreName=MX64_ID3  DataStoreElements=MX64_ID3.goal_position
  Data Store Write7 : DataStoreWrite  DataStoreName=MX64_ID5  DataStoreElements=MX64_ID5.goal_position
  Data Store Write8 : DataStoreWrite  DataStoreName=MX106_ID6  DataStoreElements=MX106_ID6.goal_position
  Data Store Write9 : DataStoreWrite  DataStoreName=MX106_ID8  DataStoreElements=MX106_ID8.goal_position
  Data Type Conversion : DataTypeConversion  OutDataTypeStr=int16
  Demux : Demux  Outputs=20
  Radians to Discrete : Gain  Gain=(4096*180)/(360*pi)  SaturateOnIntegerOverflow=on  OutDataTypeStr=Inherit: Same as input
  wires:
  Demux/3 -> Data Store Write3/1  "ID2"
  Demux/19 -> Data Store Write/1  "ID18"
  Demux/17 -> Data Store Write13/1  "ID16"
  Demux/16 -> Data Store Write18/1  "ID15"
  Demux/6 -> Data Store Write7/1  "ID5"
  Demux/10 -> Data Store Write15/1  "ID9"
  Demux/12 -> Data Store Write16/1  "ID11"
  Demux/20 -> Data Store Write1/1  "ID19"
  Demux/13 -> Data Store Write11/1  "ID12"
  Demux/15 -> Data Store Write12/1  "ID14"
  Demux/18 -> Data Store Write19/1  "ID17"
  Demux/14 -> Data Store Write17/1  "ID13"
  Demux/4 -> Data Store Write6/1  "ID3"
  Demux/1 -> Data Store Write2/1  "ID0"
  Demux/9 -> Data Store Write9/1  "ID8"
  Demux/11 -> Data Store Write10/1  "ID10"
  Demux/2 -> Data Store Write5/1  "ID1"
  Demux/7 -> Data Store Write8/1  "ID6"
  Demux/8 -> Data Store Write14/1  "ID7"
  Demux/5 -> Data Store Write4/1  "ID4"
  Constant/1 -> Add/1
  Radians to Discrete/1 -> Add/2
  Data Type Conversion/1 -> Demux/1
  Add/1 -> Data Type Conversion/1
  servo commands/1 -> Radians to Discrete/1

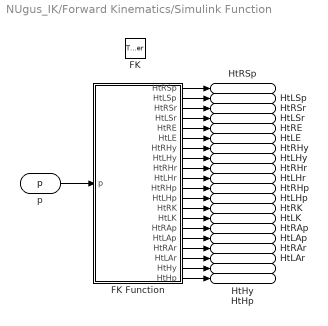
== system NUgus_IK/Forward Kinematics/Simulink Function ==
  FK : TriggerPort  TriggerType=function-call  IsSimulinkFunction=on  FunctionName=FK  FunctionVisibility=scoped  VariantControl=(inherit)
  FK Function : MATLAB Function  TreatAsAtomicUnit=on
  p : ArgIn  DisableCoverage=on  PortDimensions=[1 20]  ArgumentName=p
  HtRSp : ArgOut  DisableCoverage=on  PortDimensions=[4 4]  ArgumentName=HtRSp
  HtLSp : ArgOut  DisableCoverage=on  Port=2  PortDimensions=[4 4]  ArgumentName=HtLSp
  HtRSr : ArgOut  DisableCoverage=on  Port=3  PortDimensions=[4 4]  ArgumentName=HtRSr
  HtLSr : ArgOut  DisableCoverage=on  Port=4  PortDimensions=[4 4]  ArgumentName=HtLSr
  HtRE : ArgOut  DisableCoverage=on  Port=5  PortDimensions=[4 4]  ArgumentName=HtRE
  HtLE : ArgOut  DisableCoverage=on  Port=6  PortDimensions=[4 4]  ArgumentName=HtLE
  HtRHy : ArgOut  DisableCoverage=on  Port=7  PortDimensions=[4 4]  ArgumentName=HtRHy
  HtLHy : ArgOut  DisableCoverage=on  Port=8  PortDimensions=[4 4]  ArgumentName=HtLHy
  HtRHr : ArgOut  DisableCoverage=on  Port=9  PortDimensions=[4 4]  ArgumentName=HtRHr
  HtLHr : ArgOut  DisableCoverage=on  Port=10  PortDimensions=[4 4]  ArgumentName=HtLHr
  HtRHp : ArgOut  DisableCoverage=on  Port=11  PortDimensions=[4 4]  ArgumentName=HtRHp
  HtLHp : ArgOut  DisableCoverage=on  Port=12  PortDimensions=[4 4]  ArgumentName=HtLHp
  HtRK : ArgOut  DisableCoverage=on  Port=13  PortDimensions=[4 4]  ArgumentName=HtRK
  HtLK : ArgOut  DisableCoverage=on  Port=14  PortDimensions=[4 4]  ArgumentName=HtLK
  HtRAp : ArgOut  DisableCoverage=on  Port=15  PortDimensions=[4 4]  ArgumentName=HtRAp
  HtLAp : ArgOut  DisableCoverage=on  Port=16  PortDimensions=[4 4]  ArgumentName=HtLAp
  HtRAr : ArgOut  DisableCoverage=on  Port=17  PortDimensions=[4 4]  ArgumentName=HtRAr
  HtLAr : ArgOut  DisableCoverage=on  Port=18  PortDimensions=[4 4]  ArgumentName=HtLAr
  HtHy : ArgOut  DisableCoverage=on  Port=19  PortDimensions=[4 4]  ArgumentName=HtHy
  HtHp : ArgOut  DisableCoverage=on  Port=20  PortDimensions=[4 4]  ArgumentName=HtHp
  wires:
  p/1 -> FK Function/1(p)
  FK Function/15(HtRAp) -> HtRAp/1
  FK Function/10(HtLHr) -> HtLHr/1
  FK Function/9(HtRHr) -> HtRHr/1
  FK Function/8(HtLHy) -> HtLHy/1
  FK Function/7(HtRHy) -> HtRHy/1
  FK Function/2(HtLSp) -> HtLSp/1
  FK Function/14(HtLK) -> HtLK/1
  FK Function/3(HtRSr) -> HtRSr/1
  FK Function/6(HtLE) -> HtLE/1
  FK Function/5(HtRE) -> HtRE/1
  FK Function/1(HtRSp) -> HtRSp/1
  FK Function/16(HtLAp) -> HtLAp/1
  FK Function/17(HtRAr) -> HtRAr/1
  FK Function/19(HtHy) -> HtHy/1
  FK Function/4(HtLSr) -> HtLSr/1
  FK Function/20(HtHp) -> HtHp/1
  FK Function/11(HtRHp) -> HtRHp/1
  FK Function/12(HtLHp) -> HtLHp/1
  FK Function/13(HtRK) -> HtRK/1
  FK Function/18(HtLAr) -> HtLAr/1

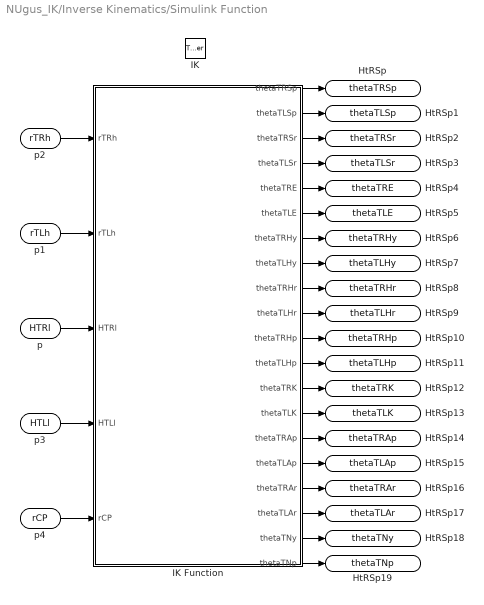
== system NUgus_IK/Inverse Kinematics/Simulink Function ==
  IK : TriggerPort  TriggerType=function-call  IsSimulinkFunction=on  FunctionName=IK  FunctionVisibility=scoped  VariantControl=(inherit)
  IK Function : MATLAB Function  TreatAsAtomicUnit=on
  p2 : ArgIn  DisableCoverage=on  PortDimensions=[1 3]  ArgumentName=rTRh
  p1 : ArgIn  DisableCoverage=on  Port=2  PortDimensions=[1 3]  ArgumentName=rTLh
  p : ArgIn  DisableCoverage=on  Port=3  PortDimensions=[4 4]  ArgumentName=HTRl
  p3 : ArgIn  DisableCoverage=on  Port=4  PortDimensions=[4 4]  ArgumentName=HTLl
  p4 : ArgIn  DisableCoverage=on  Port=5  PortDimensions=[1 3]  ArgumentName=rCP
  HtRSp : ArgOut  DisableCoverage=on  ArgumentName=thetaTRSp
  HtRSp1 : ArgOut  DisableCoverage=on  Port=2  ArgumentName=thetaTLSp
  HtRSp2 : ArgOut  DisableCoverage=on  Port=3  ArgumentName=thetaTRSr
  HtRSp3 : ArgOut  DisableCoverage=on  Port=4  ArgumentName=thetaTLSr
  HtRSp4 : ArgOut  DisableCoverage=on  Port=5  ArgumentName=thetaTRE
  HtRSp5 : ArgOut  DisableCoverage=on  Port=6  ArgumentName=thetaTLE
  HtRSp6 : ArgOut  DisableCoverage=on  Port=7  ArgumentName=thetaTRHy
  HtRSp7 : ArgOut  DisableCoverage=on  Port=8  ArgumentName=thetaTLHy
  HtRSp8 : ArgOut  DisableCoverage=on  Port=9  ArgumentName=thetaTRHr
  HtRSp9 : ArgOut  DisableCoverage=on  Port=10  ArgumentName=thetaTLHr
  HtRSp10 : ArgOut  DisableCoverage=on  Port=11  ArgumentName=thetaTRHp
  HtRSp11 : ArgOut  DisableCoverage=on  Port=12  ArgumentName=thetaTLHp
  HtRSp12 : ArgOut  DisableCoverage=on  Port=13  ArgumentName=thetaTRK
  HtRSp13 : ArgOut  DisableCoverage=on  Port=14  ArgumentName=thetaTLK
  HtRSp14 : ArgOut  DisableCoverage=on  Port=15  ArgumentName=thetaTRAp
  HtRSp15 : ArgOut  DisableCoverage=on  Port=16  ArgumentName=thetaTLAp
  HtRSp16 : ArgOut  DisableCoverage=on  Port=17  ArgumentName=thetaTRAr
  HtRSp17 : ArgOut  DisableCoverage=on  Port=18  ArgumentName=thetaTLAr
  HtRSp18 : ArgOut  DisableCoverage=on  Port=19  ArgumentName=thetaTNy
  HtRSp19 : ArgOut  DisableCoverage=on  Port=20  ArgumentName=thetaTNp
  wires:
  p/1 -> IK Function/3(HTRl)
  p1/1 -> IK Function/2(rTLh)
  p2/1 -> IK Function/1(rTRh)
  p3/1 -> IK Function/4(HTLl)
  p4/1 -> IK Function/5(rCP)
  IK Function/1(thetaTRSp) -> HtRSp/1
  IK Function/2(thetaTLSp) -> HtRSp1/1
  IK Function/3(thetaTRSr) -> HtRSp2/1
  IK Function/4(thetaTLSr) -> HtRSp3/1
  IK Function/5(thetaTRE) -> HtRSp4/1
  IK Function/6(thetaTLE) -> HtRSp5/1
  IK Function/7(thetaTRHy) -> HtRSp6/1
  IK Function/8(thetaTLHy) -> HtRSp7/1
  IK Function/9(thetaTRHr) -> HtRSp8/1
  IK Function/10(thetaTLHr) -> HtRSp9/1
  IK Function/11(thetaTRHp) -> HtRSp10/1
  IK Function/12(thetaTLHp) -> HtRSp11/1
  IK Function/13(thetaTRK) -> HtRSp12/1
  IK Function/14(thetaTLK) -> HtRSp13/1
  IK Function/15(thetaTRAp) -> HtRSp14/1
  IK Function/16(thetaTLAp) -> HtRSp15/1
  IK Function/17(thetaTRAr) -> HtRSp16/1
  IK Function/18(thetaTLAr) -> HtRSp17/1
  IK Function/19(thetaTNy) -> HtRSp18/1
  IK Function/20(thetaTNp) -> HtRSp19/1

== system NUgus_IK/NUgus/head ==
  Inertia : sm_lib/Body Elements/Inertia  InertiaType=Custom  Mass=0.419  MassUnits=kg  CenterOfMass=[0, 0, 0]  CenterOfMassUnits=m  MomentsOfInertia=[0.00522954263224, 0.00427382206022, 0.00333363205267]  MomentsOfInertiaUnits=kg*m^2  ProductsOfInertia=[2.26332170851e-07, -7.85419377514e-05, 8.06868913029e-07]  ProductsOfInertiaUnits=kg*m^2  GraphicType=None  MarkerShape=Inertia  MarkerSize=20  GraphicVisPropType=SimpleVisualProperties  GraphicDiffuseColor=[0.5 0.5 0.5]  GraphicSpecularColor=[0.5 0.5 0.5 1.0]  GraphicAmbientColor=[0.15 0.15 0.15 1.0]  GraphicEmissiveColor=[0.0 0.0 0.0 1.0]  GraphicShininess=75  GraphicOpacity=1.0
  InertiaOriginTransform : sm_lib/Frames and Transforms/Rigid Transform  TranslationMethod=Cartesian  TranslationStandardOffset=0  TranslationLengthUnit=m  TranslationStandardAxis=+Z  TranslationCartesianOffset=[-0.002841 -0.003496 0.064412]  TranslationROffset=0  TranslationROffsetUnits=m  TranslationZOffset=0  TranslationZOffsetUnits=m  TranslationThetaOffset=0  TranslationThetaOffsetUnits=deg  RotationMethod=RotationSequence  RotationAngleUnits=deg  RotationStandardAxis=+Z  RotationAngle=0.0  RotationArbitraryAxis=[0 0 1]  FollAlignAxisA=+X  BaseAlignAxisA=+Y  FollAlignAxisB=+Y  BaseAlignAxisB=+Z  RotationSequenceAxes=BaseAxes  RotationSequence=XYZ  RotationSequenceAngles=[0, 0, 0]  RotationSequenceAnglesUnits=rad  RotationMatrix=[1 0 0; 0 1 0; 0 0 1]
  ReferenceFrame : sm_lib/Frames and Transforms/Reference Frame
  head_pitch_AxisInvTransform : sm_lib/Frames and Transforms/Rigid Transform  TranslationMethod=Cartesian  TranslationStandardOffset=0  TranslationLengthUnit=m  TranslationStandardAxis=+Z  TranslationCartesianOffset=[0, 0, 0]  TranslationROffset=0  TranslationROffsetUnits=m  TranslationZOffset=0  TranslationZOffsetUnits=m  TranslationThetaOffset=0  TranslationThetaOffsetUnits=deg  RotationMethod=ArbitraryAxis  RotationAngleUnits=rad  RotationStandardAxis=+Z  RotationAngle=1.570796326794897  RotationArbitraryAxis=[-0, 1, 0]  FollAlignAxisA=+X  BaseAlignAxisA=+Y  FollAlignAxisB=+Y  BaseAlignAxisB=+Z  RotationSequenceAxes=FollowerAxes  RotationSequence=XYX  RotationSequenceAngles=[0 0 0]  RotationSequenceAnglesUnits=deg  RotationMatrix=[1 0 0; 0 1 0; 0 0 1]
  head_visual : sm_lib/Body Elements/Solid  InertiaType=Custom  Mass=0  MassUnits=kg  CenterOfMass=[0, 0, 0]  CenterOfMassUnits=m  MomentsOfInertia=[0, 0, 0]  MomentsOfInertiaUnits=kg*m^2  ProductsOfInertia=[0, 0, 0]  ProductsOfInertiaUnits=kg*m^2  DensityBased=on  Density=1000  DensityUnits=kg/m^3  DoExposeReferenceFrame=on  SerializedFrames=<Frames/>  GraphicType=FromGeometry  MarkerShape=Sphere  MarkerSize=10  GraphicVisPropType=SimpleVisualProperties  GraphicDiffuseColor=[0.5, 0.5, 0.5]  GraphicSpecularColor=[0.5 0.5 0.5 1.0]  GraphicAmbientColor=[0.15 0.15 0.15 1.0]  GraphicEmissiveColor=[0.0 0.0 0.0 1.0]  GraphicShininess=75  GraphicOpacity=1  GeometryShape=FromFile  RectangleSize=[1 1]  RectangleSizeUnits=m  BrickDimensions=[1 1 1]  BrickDimensionUnits=m  CylinderRadius=1  CylinderRadiusUnits=m  CylinderLength=1  CylinderLengthUnits=m  SphereRadius=1  SphereRadiusUnits=m  EllipsoidRadii=[1 1 1]  EllipsoidRadiiUnits=m  ExtrusionCrossSection=[1 1; -1 1; -1 -1; 1 -1]  ExtrusionCrossSectionUnits=m  ExtrusionLength=1  ExtrusionLengthUnits=m  PolygonNumSides=3  PolygonOuterRadius=1  PolygonOuterRadiusUnits=m  ExtGeomFileType=STL  ExtGeomFileName=mesh/head.stl  ExtGeomFileUnits=m  RevolutionCrossSection=[1 1; 1 -1; 2 -1; 2 1]  RevolutionCrossSectionUnits=m  RevolutionExtent=Full  RevolutionAngle=180  RevolutionAngleUnits=deg
  head_visualOriginTransform : sm_lib/Frames and Transforms/Rigid Transform  TranslationMethod=Cartesian  TranslationStandardOffset=0  TranslationLengthUnit=m  TranslationStandardAxis=+Z  TranslationCartesianOffset=[0, 0, 0]  TranslationROffset=0  TranslationROffsetUnits=m  TranslationZOffset=0  TranslationZOffsetUnits=m  TranslationThetaOffset=0  TranslationThetaOffsetUnits=deg  RotationMethod=RotationSequence  RotationAngleUnits=deg  RotationStandardAxis=+Z  RotationAngle=0.0  RotationArbitraryAxis=[0 0 1]  FollAlignAxisA=+X  BaseAlignAxisA=+Y  FollAlignAxisB=+Y  BaseAlignAxisB=+Z  RotationSequenceAxes=BaseAxes  RotationSequence=XYZ  RotationSequenceAngles=[0, 0, 0]  RotationSequenceAnglesUnits=rad  RotationMatrix=[1 0 0; 0 1 0; 0 0 1]
  F : PMIOPort  Side=Left
  connections:
  Inertia/RConn1 -- InertiaOriginTransform/RConn1
  ReferenceFrame/RConn1 -- InertiaOriginTransform/LConn1 -- head_pitch_AxisInvTransform/LConn1 -- head_visualOriginTransform/LConn1
  head_pitch_AxisInvTransform/RConn1 -- F/RConn1
  head_visual/RConn1 -- head_visualOriginTransform/RConn1

== system NUgus_IK/NUgus/head_pitch ==
  Data Store Read : DataStoreRead  DataStoreName=MX64_ID19  DataStoreElements=MX64_ID19.CW_angle_limit#MX64_ID19.CCW_angle_limit#MX64_ID19.torque_enable#MX64_ID19.D_gain#MX64_ID19.I_gain#MX64_ID19.P_gain#MX64_ID19.goal_position#MX64_ID19.moving_speed#MX64_ID19.torque_limit
  Data Store Write : DataStoreWrite  DataStoreName=MX64_ID19  DataStoreElements=MX64_ID19.present_position#MX64_ID19.present_speed#MX64_ID19.present_load#MX64_ID19.moving#MX64_ID19.pwm
  Joint : sm_lib/Joints/Revolute Joint  SenseConstraintForce=off  SenseConstraintForceX=off  SenseConstraintForceY=off  SenseConstraintForceZ=off  SenseConstraintTorque=off  SenseConstraintTorqueX=off  SenseConstraintTorqueY=off  SenseConstraintTorqueZ=off  SenseTotalForce=off  SenseTotalForceX=off  SenseTotalForceY=off  SenseTotalForceZ=off  SenseTotalTorque=off  SenseTotalTorqueX=off  SenseTotalTorqueY=off  SenseTotalTorqueZ=off  CompositeWrenchDir=FollowerOnBase  CompositeWrenchFrame=BaseFrame  EquilibriumPosition=0  EquilibriumPositionUnits=deg  SpringStiffness=0  SpringStiffnessUnits=N*m/deg  DampingCoefficient=MX64_lub_friction  DampingCoefficientUnits=N*m/(rad/s)  TorqueActuationMode=InputTorque  MotionActuationMode=ComputedMotion  SensePosition=on  SenseVelocity=on  SenseAcceleration=off  SenseTorqueForce=off  PositionTargetSpecify=on  PositionTargetPriority=High  PositionTargetValue=MX64_init_position  PositionTargetValueUnits=rad  VelocityTargetSpecify=on  VelocityTargetPriority=High  VelocityTargetValue=MX64_init_speed  VelocityTargetValueUnits=rad/s
  Model : ModelReference  ModelNameDialog=MX64  SimulationMode=Normal  ModelReferenceVersion=1.25
  Position : nesl_utility/PS-Simulink Converter  PhysicalDomain=network_engine_domain  SubClassName=ps_output  LeftPortType=input  RightPortType=output  PseudoPeriodic=off  Frequencies=[]  Unit=rad  AffineConversion=off
  Simulink-PS Converter : nesl_utility/Simulink-PS Converter  PhysicalDomain=network_engine_domain  SubClassName=ps_input  LeftPortType=input  RightPortType=output  PseudoPeriodic=off  Frequencies=[]  NoiseDistribution=none  NoiseParameters=[]  Unit=N*m  AffineConversion=off  FilteringAndDerivatives=zero  SimscapeFilterOrder=1  InputFilterTimeConstant=0.001  UdotUserProvided=0
  Speed : nesl_utility/PS-Simulink Converter  PhysicalDomain=network_engine_domain  SubClassName=ps_output  LeftPortType=input  RightPortType=output  PseudoPeriodic=off  Frequencies=[]  Unit=rad/s  AffineConversion=off
  B : PMIOPort  Side=Left
  F : PMIOPort  Port=2  Side=Right
  wires:
  Speed/1 -> Model/1
  Position/1 -> Model/2
  Data Store Read/1 -> Model/3
  Data Store Read/2 -> Model/4
  Data Store Read/3 -> Model/5
  Data Store Read/4 -> Model/6
  Data Store Read/5 -> Model/7
  Data Store Read/6 -> Model/8
  Data Store Read/7 -> Model/9
  Data Store Read/8 -> Model/10
  Data Store Read/9 -> Model/11
  Model/2 -> Data Store Write/1
  Model/3 -> Data Store Write/2
  Model/4 -> Data Store Write/3
  Model/5 -> Data Store Write/4
  Model/6 -> Data Store Write/5
  Model/1 -> Simulink-PS Converter/1
  connections:
  Joint/RConn1 -- F/RConn1
  Joint/LConn1 -- B/RConn1
  Joint/LConn2 -- Simulink-PS Converter/RConn1
  Joint/RConn3 -- Speed/LConn1
  Joint/RConn2 -- Position/LConn1
